simulink library "Utilities"  (R2024a)
settings: Solver=VariableStepAuto  StartTime=0.0  StopTime=10.0  RelTol=1e-3
values from neighbouring files (symbols this model uses):
  StateCAN : value not decoded    [Utilities.sldd]
undefined symbols (not defined in the file or in its folder): enum2Raptor, raptor_xcp_function
libraries: simulink x5, Raptor_lib x4
settings Model: Creator=serga  LastModifiedBy=serga
settings OptimizationCC: ReuseModelBlockBuffer=off
settings RTWCC: GPUComputeCapability=3.5

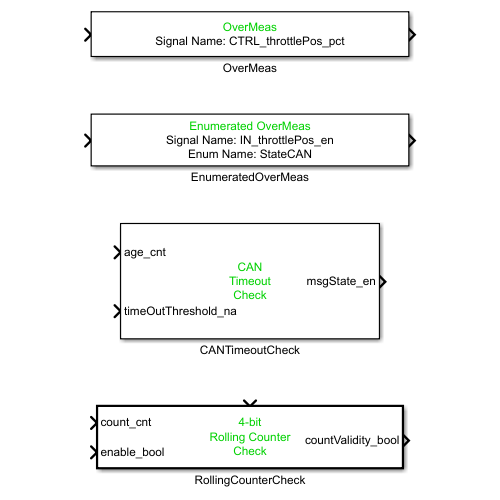
[thumbnail: Simulink's stored preview of the top-level diagram]
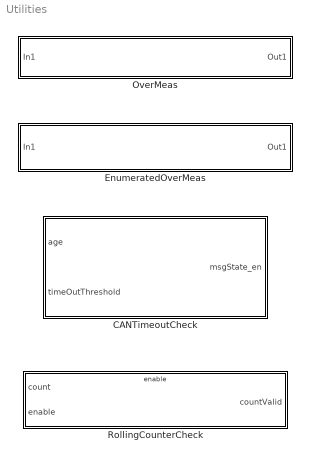
== system Utilities ==
  CANTimeoutCheck : Subsystem
      mask Display:
      | color('green')
      | disp('CAN\nTimeout\nCheck')
      | color('black')
      | port_label('input', 1, 'age_cnt');
      | port_label('input', 2, 'timeOutThreshold_na');
      | port_label('output', 1, 'msgState_en')
  EnumeratedOverMeas : Subsystem  mask{sigName='IN_throttlePos_en', enumName='StateCAN'}
      mask prompts: sigName "Signal Name"; enumName "Enumeration Name"
      mask init:
      | set_param([gcb '/Data Type Conversion1'],'OutDataTypeStr',['Enum:' enumName]);
      |     try
      |         p = get_param(gcb, 'PortHandles');
      |         l = get_param(p.Outport, 'Line');
      |         set_param(l, 'Name', sigName);
      |     end
      mask Display:
      | color('green')
      | disp('Enumerated OverMeas\n\n')
      | color('black')
      | disp(['Signal Name: ' sigName])
      | disp(['\n\nEnum Name: ' enumName])
  OverMeas : Subsystem  mask{sigName='CTRL_throttlePos_pct', min=-inf, max=inf}
      mask prompts: sigName "Signal Name"; min "Minimum"; max "Maximum"
      mask init:
      | %labels outports as the signal name
      |     try
      |         p = get_param(gcb, 'PortHandles');
      |         l = get_param(p.Outport, 'Line');
      |         set_param(l, 'Name', sigName);
      |     end
      mask Display:
      | color('green')
      | disp('OverMeas\n')
      | color('black')
      | disp(['\nSignal Name: ' sigName])
  RollingCounterCheck : Subsystem  TreatAsAtomicUnit=on
      mask Display:
      | color('green')
      | disp('4-bit\nRolling Counter\nCheck')
      | color('black')
      | port_label('input', 1, 'count_cnt');
      | port_label('input', 2, 'enable_bool');
      | port_label('output', 1, 'countValidity_bool')

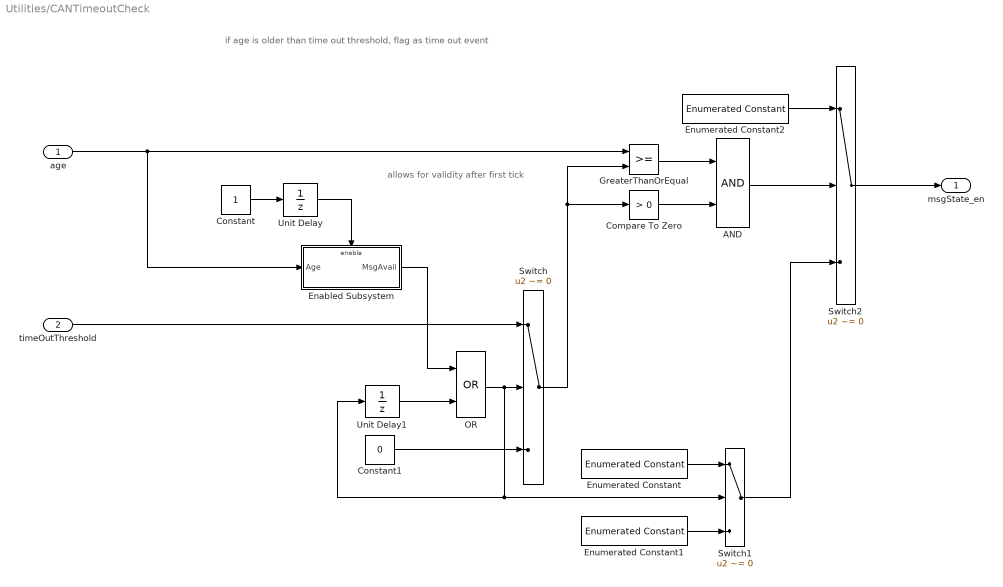
== system Utilities/CANTimeoutCheck ==
  note: if age is older than time out threshold, flag as time out event
  note: allows for validity after first tick
  age : Inport
  timeOutThreshold : Inport  Port=2
  AND : Logic  AllPortsSameDT=off  OutDataTypeStr=boolean
  Compare To Zero : simulink/Logic and Bit Operations/Compare To Zero  relop=>  OutDataTypeStr=boolean
  Constant : Constant  OutDataTypeStr=boolean
  Constant1 : Constant  Value=0  OutDataTypeStr=boolean
  Enabled Subsystem : Subsystem  TreatAsAtomicUnit=on
  Enumerated Constant : simulink/Sources/Enumerated Constant  OutDataTypeStr=Enum: StateCAN  Value=StateCAN.Normal  SampleTime=inf
  Enumerated Constant1 : simulink/Sources/Enumerated Constant  OutDataTypeStr=Enum: StateCAN  Value=StateCAN.NotReceived  SampleTime=inf
  Enumerated Constant2 : simulink/Sources/Enumerated Constant  OutDataTypeStr=Enum: StateCAN  Value=StateCAN.TimedOut  SampleTime=inf
  GreaterThanOrEqual : RelationalOperator  OutDataTypeStr=boolean  RndMeth=Simplest  InputSameDT=off
  OR : Logic  Operator=OR  AllPortsSameDT=off  OutDataTypeStr=boolean
  Switch : Switch  Criteria=u2 ~= 0  SaturateOnIntegerOverflow=off  InputSameDT=off
  Switch1 : Switch  Criteria=u2 ~= 0  SaturateOnIntegerOverflow=off  InputSameDT=off
  Switch2 : Switch  Criteria=u2 ~= 0  SaturateOnIntegerOverflow=off  InputSameDT=off
  Unit Delay : UnitDelay  SampleTime=-1  HasFrameUpgradeWarning=on
  Unit Delay1 : UnitDelay  SampleTime=-1  HasFrameUpgradeWarning=on
  msgState_en : Outport
  wires:
  Constant/1 -> Unit Delay/1
  Unit Delay/1 -> Enabled Subsystem/Enable
  age/1 -> GreaterThanOrEqual/1, Enabled Subsystem/1(Age)
  timeOutThreshold/1 -> Switch/1
  OR/1 -> Unit Delay1/1, Switch1/2, Switch/2
  Enabled Subsystem/1(MsgAvail) -> OR/1
  Unit Delay1/1 -> OR/2
  Enumerated Constant/1 -> Switch1/1
  Enumerated Constant1/1 -> Switch1/3
  Constant1/1 -> Switch/3
  Switch/1 -> GreaterThanOrEqual/2, Compare To Zero/1
  GreaterThanOrEqual/1 -> AND/1
  Compare To Zero/1 -> AND/2
  AND/1 -> Switch2/2
  Switch2/1 -> msgState_en/1
  Enumerated Constant2/1 -> Switch2/1
  Switch1/1 -> Switch2/3

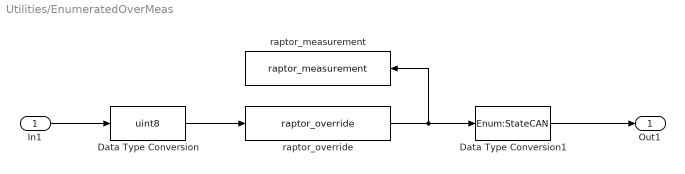
== system Utilities/EnumeratedOverMeas ==
  In1 : Inport
  Data Type Conversion : DataTypeConversion  OutDataTypeStr=uint8  SaturateOnIntegerOverflow=off  RndMeth=Floor
  Data Type Conversion1 : DataTypeConversion  OutDataTypeStr=Enum:StateCAN  SaturateOnIntegerOverflow=off  RndMeth=Floor
  raptor_measurement : Raptor_lib/Data Storage/raptor_measurement  paramName=sigName  nameSource=Parameter  calDispType=Enumeration  calEnum=enum2Raptor(enumName)  calGain=1.0  calOffset=0.0  calMax=max  calMin=min  calFormat='-1'  calUnit=''  calHelp=''  calAccess=1  calFunction=raptor_xcp_function(gcb)  calVisible=on
      settings: SourceProductName=Raptor
  raptor_override : Raptor_lib/Data Storage/raptor_override  paramName=sigName  nameSource=Parameter  measurement=None  calDispType=Enumeration  calEnum=enum2Raptor(enumName)  calGain=1.0  calOffset=0.0  calMax=max  calMin=min  calFormat='-1'  calUnit=''  calHelp=''  calAccess=1  calFunction="[raptor_xcp_function(gcb) '|'  'Override']"
      settings: SourceProductName=Raptor
  Out1 : Outport
  wires:
  In1/1 -> Data Type Conversion/1
  Data Type Conversion/1 -> raptor_override/1
  raptor_override/1 -> Data Type Conversion1/1, raptor_measurement/1
  Data Type Conversion1/1 -> Out1/1

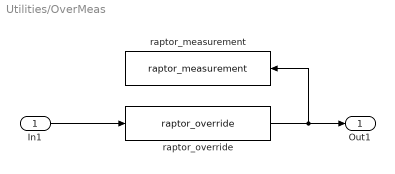
== system Utilities/OverMeas ==
  In1 : Inport
  raptor_measurement : Raptor_lib/Data Storage/raptor_measurement  paramName=sigName  nameSource=Parameter  calDispType=Number  calEnum={'False', 'True'}  calGain=1.0  calOffset=0.0  calMax=max  calMin=min  calFormat='-1'  calUnit=''  calHelp=''  calAccess=1  calFunction=raptor_xcp_function(gcb)  calVisible=on
      settings: SourceProductName=Raptor
  raptor_override : Raptor_lib/Data Storage/raptor_override  paramName=sigName  nameSource=Parameter  measurement=None  calDispType=Number  calEnum={'False', 'True'}  calGain=1.0  calOffset=0.0  calMax=max  calMin=min  calFormat='-1'  calUnit=''  calHelp=''  calAccess=1  calFunction="[raptor_xcp_function(gcb) '|'  'Override']"
      settings: SourceProductName=Raptor
  Out1 : Outport
  wires:
  In1/1 -> raptor_override/1
  raptor_override/1 -> raptor_measurement/1, Out1/1

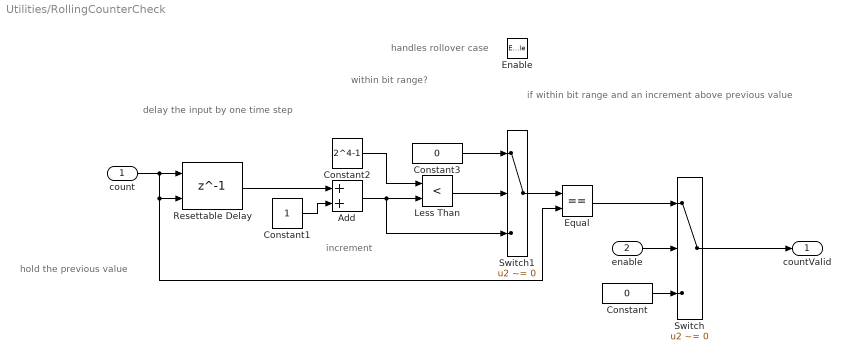
== system Utilities/RollingCounterCheck ==
  note: handles rollover case
  note: if within bit range and an increment above previous value
  note: within bit range?
  note: increment
  note: hold the previous value
  note: delay the input by one time step
  count : Inport
  enable : Inport  Port=2
  Enable : EnablePort
  Add : Sum
  Constant : Constant  Value=0  OutDataTypeStr=boolean
  Constant1 : Constant
  Constant2 : Constant  Value=2^4-1
  Constant3 : Constant  Value=0  OutDataTypeStr=boolean
  Equal : RelationalOperator  Operator===  OutDataTypeStr=boolean  RndMeth=Simplest  InputSameDT=off
  Less Than : RelationalOperator  Operator=<  OutDataTypeStr=boolean  RndMeth=Simplest  InputSameDT=off
  Resettable Delay : Delay  DelayLength=1  InitialConditionSource=Input port
      settings: InputPortMap=u0,p4
  Switch : Switch  Criteria=u2 ~= 0  SaturateOnIntegerOverflow=off  InputSameDT=off
  Switch1 : Switch  Criteria=u2 ~= 0  SaturateOnIntegerOverflow=off  InputSameDT=off
  countValid : Outport
  wires:
  count/1 -> Resettable Delay/2, Equal/2, Resettable Delay/1
  enable/1 -> Switch/2
  Switch/1 -> countValid/1
  Constant/1 -> Switch/3
  Resettable Delay/1 -> Add/1
  Add/1 -> Less Than/2, Switch1/3
  Constant2/1 -> Less Than/1
  Less Than/1 -> Switch1/2
  Constant3/1 -> Switch1/1
  Switch1/1 -> Equal/1
  Equal/1 -> Switch/1
  Constant1/1 -> Add/2

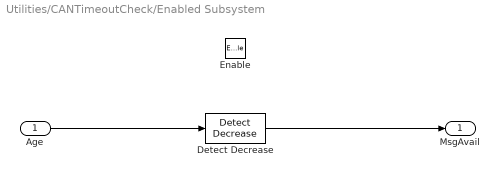
== system Utilities/CANTimeoutCheck/Enabled Subsystem ==
  Age : Inport
  Enable : EnablePort
  Detect Decrease : simulink/Logic and Bit Operations/Detect Decrease  vinit=1  OutDataTypeStr=boolean
  MsgAvail : Outport
  wires:
  Age/1 -> Detect Decrease/1
  Detect Decrease/1 -> MsgAvail/1
